simulink model "stewartplatform"  (R2019b)
settings: Solver=VariableStepAuto  StartTime=0.0  StopTime=34  RelTol=1e-3
model workspace (MAT data in the model file):
  AL = [69.992  30  41.1926948051; 60.9767621135  45.6148500617  41.1926948051; -60.9767621135  45.6148500617  41.1926948051; -69.992  30  41.1926948051; -9.01523788647  -75.6148500617  41.1926948051; 9.01523788647  -75.6148500617  41.1926948051]
  Alpha = [0.526894789881 2.61469786371 0.526894789881 2.61469786371 0.526894789881 2.61469786371]
  Alpha_ = [0.52689 2.6147 0.52689 2.6147 0.52689 2.6147]
  R = 71.492
  d = 58
  l = 1.5
  out = Simulink.SimulationOutput
  out.Data.tout = [0 3.15544362088e-30 0.00033203125 0.000660386534642 0.0011111273553 0.00167537750091 0.00236799304842 0.00321669373171 0.00427694118459 0.00567437280072 0.00710195631181 0.00848302964009 ... (1098 elements, 1098x1)]
  out.Metadata = Simulink.SimulationMetadata
  out.Metadata.ModelInfo.ModelName = 'stuartplatform'
  out.Metadata.ModelInfo.ModelVersion = '1.33'
  out.Metadata.ModelInfo.ModelFilePath = 'C:\DEV\stuartplatform\stuartplatform.slx'
  out.Metadata.ModelInfo.UserID = 'SMART PC'
  out.Metadata.ModelInfo.MachineName = 'ROBO'
  out.Metadata.ModelInfo.Platform = 'PCWIN64'
  out.Metadata.ModelInfo.ModelStructuralChecksum = [1978751953; 3150765780; 824817462; 4061112088]
  out.Metadata.ModelInfo.SimulationMode = 'normal'
  out.Metadata.ModelInfo.StartTime = 0
  out.Metadata.ModelInfo.StopTime = 1.68393954484
  out.Metadata.ModelInfo.SolverInfo.Type = 'Variable-Step'
  out.Metadata.ModelInfo.SolverInfo.Solver = 'ode45'
  out.Metadata.ModelInfo.SolverInfo.MaxStepSize = 0.68
  out.Metadata.ModelInfo.SimulinkVersion.Name = 'Simulink'
  out.Metadata.ModelInfo.SimulinkVersion.Version = '10.0'
  out.Metadata.ModelInfo.SimulinkVersion.Release = '(R2019b)'
  out.Metadata.ModelInfo.SimulinkVersion.Date = '18-Jul-2019'
  out.Metadata.ModelInfo.LoggingInfo.LoggingToFile = 'off'
  out.Metadata.TimingInfo.WallClockTimestampStart = '2020-06-21 19:02:22'
  out.Metadata.TimingInfo.WallClockTimestampStop = '2020-06-21 19:02:29'
  out.Metadata.TimingInfo.InitializationElapsedWallTime = 2.0463991
  out.Metadata.TimingInfo.ExecutionElapsedWallTime = 4.395282
  out.Metadata.TimingInfo.TerminationElapsedWallTime = 0.0061196
  out.Metadata.TimingInfo.TotalElapsedWallTime = 6.4478007
  out.Metadata.ExecutionInfo.StopEvent = 'StopCommand'
  out.Metadata.ExecutionInfo.StopEventSource = []
  out.Metadata.ExecutionInfo.StopEventDescription = 'Stop command issued at time 1.68394'
  out.Metadata.ExecutionInfo.ErrorDiagnostic = []
  out.Metadata.ExecutionInfo.WarningDiagnostics = struct([])
  out.Metadata.AppInfo = struct()
  p = 25
  q = 5.79
  r = 17.5
  rotangle = 1.0471975512
  smbData.shaping_wheels.Left.RigidTransform.angles = [1.57079632679 0.523598775598 0]
  smbData.shaping_wheels.Left.RigidTransform.ID = ''
  smbData.side_servo_SG90(1).Left.RigidTransform.angles = [1.57079632679 0 -1.0471975512]
  smbData.side_servo_SG90(1).Left.RigidTransform.translation = [59.315811956; 45.5; 34.246]
  smbData.side_servo_SG90(1).Left.RigidTransform.ID = ''
  smbData.side_servo_SG90(2).Left.RigidTransform.angles = [1.57079632679 0 -2.09439510239]
  smbData.side_servo_SG90(2).Left.RigidTransform.translation = [59.315811956; 45.5; -34.246]
  smbData.side_servo_SG90(2).Left.RigidTransform.ID = ''
  smbData.side_servo_SG90(3).Left.RigidTransform.angles = [1.57079632679 0 -3.14159265359]
  smbData.side_servo_SG90(3).Left.RigidTransform.translation = [8.38785085672e-15; 45.5; -68.492]
  smbData.side_servo_SG90(3).Left.RigidTransform.ID = ''
  smbData.side_servo_SG90(4).Left.RigidTransform.angles = [1.57079632679 0 -4.18879020479]
  smbData.side_servo_SG90(4).Left.RigidTransform.translation = [-59.315811956; 45.5; -34.246]
  smbData.side_servo_SG90(4).Left.RigidTransform.ID = ''
  smbData.side_servo_SG90(5).Left.RigidTransform.angles = [1.57079632679 0 -5.23598775598]
  smbData.side_servo_SG90(5).Left.RigidTransform.translation = [-59.315811956; 45.5; 34.246]
  smbData.side_servo_SG90(5).Left.RigidTransform.ID = ''
  smbData.side_servo_SG90(6).Left.RigidTransform.angles = [1.57079632679 0 -6.28318530718]
  smbData.side_servo_SG90(6).Left.RigidTransform.translation = [-1.67757017134e-14; 45.5; 68.492]
  smbData.side_servo_SG90(6).Left.RigidTransform.ID = ''
  smbData.servo_SG90(1).Left.RigidTransform.angles = [0 0 0]
  smbData.servo_SG90(1).Right.RigidTransform.angles = [-1.57079632679 0 0]
  smbData.servo_SG90(1).Right.RigidTransform.translation = [-5.79; 11.5; 0]
  smbData.servo_SG90(1).Right.RigidTransform.ID = ''
  smbData.servo_SG90(2).Left.RigidTransform.angles = [0 3.14159265359 0]
  smbData.servo_SG90(2).Right.RigidTransform.angles = [-1.57079632679 0 3.14159265359]
  smbData.servo_SG90(2).Right.RigidTransform.translation = [-5.79; 11.5; 0]
  smbData.servo_SG90(2).Right.RigidTransform.ID = ''
  smbData.servo_SG90(3).Left.RigidTransform.angles = [0 6.28318530718 0]
  smbData.servo_SG90(3).Right.RigidTransform.angles = [-1.57079632679 0 6.28318530718]
  smbData.servo_SG90(3).Right.RigidTransform.translation = [-5.79; 11.5; 0]
  smbData.servo_SG90(3).Right.RigidTransform.ID = ''
  smbData.servo_SG90(4).Left.RigidTransform.angles = [0 9.42477796077 0]
  smbData.servo_SG90(4).Right.RigidTransform.angles = [-1.57079632679 0 9.42477796077]
  smbData.servo_SG90(4).Right.RigidTransform.translation = [-5.79; 11.5; 0]
  smbData.servo_SG90(4).Right.RigidTransform.ID = ''
  smbData.servo_SG90(5).Left.RigidTransform.angles = [0 12.5663706144 0]
  smbData.servo_SG90(5).Right.RigidTransform.angles = [-1.57079632679 0 12.5663706144]
  smbData.servo_SG90(5).Right.RigidTransform.translation = [-5.79; 11.5; 0]
  smbData.servo_SG90(5).Right.RigidTransform.ID = ''
  smbData.servo_SG90(6).Left.RigidTransform.angles = [0 15.7079632679 0]
  smbData.servo_SG90(6).Right.RigidTransform.angles = [-1.57079632679 0 15.7079632679]
  smbData.servo_SG90(6).Right.RigidTransform.translation = [-5.79; 11.5; 0]
  smbData.servo_SG90(6).Right.RigidTransform.ID = ''
  smbData.link_active(1).Left.RigidTransform.angles = [1.57079632679 0 0]
  smbData.link_active(1).Left.RigidTransform.ID = ''
  smbData.link_active(1).Right.RigidTransform.angles = [1.57079632679 0 3.14159265359]
  smbData.link_active(1).Right.RigidTransform.translation = [-15.1842023169; 16.5; 0]
  smbData.link_active(1).Right.RigidTransform.ID = ''
  smbData.link_active(2).Left.RigidTransform.angles = [1.57079632679 0 0]
  smbData.link_active(2).Left.RigidTransform.ID = ''
  smbData.link_active(2).Right.RigidTransform.angles = [1.57079632679 0 6.28318530718]
  smbData.link_active(2).Right.RigidTransform.translation = [-15.1842023169; 16.5; 0]
  smbData.link_active(2).Right.RigidTransform.ID = ''
  smbData.link_active(3).Left.RigidTransform.angles = [1.57079632679 0 0]
  smbData.link_active(3).Left.RigidTransform.ID = ''
  smbData.link_active(3).Right.RigidTransform.angles = [1.57079632679 0 9.42477796077]
  smbData.link_active(3).Right.RigidTransform.translation = [-15.1842023169; 16.5; 0]
  smbData.link_active(3).Right.RigidTransform.ID = ''
  smbData.link_active(4).Left.RigidTransform.angles = [1.57079632679 0 0]
  smbData.link_active(4).Left.RigidTransform.ID = ''
  smbData.link_active(4).Right.RigidTransform.angles = [1.57079632679 0 12.5663706144]
  smbData.link_active(4).Right.RigidTransform.translation = [-15.1842023169; 16.5; 0]
  smbData.link_active(4).Right.RigidTransform.ID = ''
  smbData.link_active(5).Left.RigidTransform.angles = [1.57079632679 0 0]
  smbData.link_active(5).Left.RigidTransform.ID = ''
  smbData.link_active(5).Right.RigidTransform.angles = [1.57079632679 0 15.7079632679]
  smbData.link_active(5).Right.RigidTransform.translation = [-15.1842023169; 16.5; 0]
  smbData.link_active(5).Right.RigidTransform.ID = ''
  smbData.link_active(6).Left.RigidTransform.angles = [1.57079632679 0 0]
  smbData.link_active(6).Left.RigidTransform.ID = ''
  smbData.link_active(6).Right.RigidTransform.angles = [1.57079632679 0 18.8495559215]
  smbData.link_active(6).Right.RigidTransform.translation = [-15.1842023169; 16.5; 0]
  smbData.link_active(6).Right.RigidTransform.ID = ''
  smbData.joint_universal_between_axises_30 = [0 8.7 0]
  smbData.joint_universal_between_axises_15 = [0 8.7 0]
  smbData.joint_universal_30(1).Right.RigidTransform.angles = [0 0 0.520302761315]
  smbData.joint_universal_30(2).Right.RigidTransform.angles = [0 0 -0.520302761315]
  smbData.joint_universal_30(3).Right.RigidTransform.angles = [0 0 0.520302761315]
  smbData.joint_universal_30(4).Right.RigidTransform.angles = [0 0 -0.520302761315]
  smbData.joint_universal_30(5).Right.RigidTransform.angles = [0 0 0.520302761315]
  smbData.joint_universal_30(6).Right.RigidTransform.angles = [0 0 -0.520302761315]
  smbData.joint_universal_cube(1).Left.RigidTransform.angles = [0 0 -0.0054062780322]
  smbData.joint_universal_cube(1).Right.RigidTransform.angles = [0 1.57079632679 0.474503156818]
  smbData.joint_universal_cube(2).Left.RigidTransform.angles = [0 0 0.00540627803224]
  smbData.joint_universal_cube(2).Right.RigidTransform.angles = [0 1.57079632679 0.474503156818]
  smbData.joint_universal_cube(3).Left.RigidTransform.angles = [0 0 -0.0054062780322]
  smbData.joint_universal_cube(3).Right.RigidTransform.angles = [0 1.57079632679 0.474503156818]
  smbData.joint_universal_cube(4).Left.RigidTransform.angles = [0 0 0.00540627803224]
  smbData.joint_universal_cube(4).Right.RigidTransform.angles = [0 1.57079632679 0.474503156818]
  smbData.joint_universal_cube(5).Left.RigidTransform.angles = [0 0 -0.0054062780322]
  smbData.joint_universal_cube(5).Right.RigidTransform.angles = [0 1.57079632679 0.474503156818]
  smbData.joint_universal_cube(6).Left.RigidTransform.angles = [0 0 0.0054062780322]
  smbData.joint_universal_cube(6).Right.RigidTransform.angles = [0 1.57079632679 0.474503156818]
  smbData.joint_universal_15(1).Left.RigidTransform.angles = [0 0 -3.14159265359]
  smbData.joint_universal_15(1).Right.RigidTransform.angles = [3.14159265359 3.14159265359 0]
  smbData.joint_universal_15(2).Left.RigidTransform.angles = [0 0 -3.14159265359]
  smbData.joint_universal_15(2).Right.RigidTransform.angles = [3.14159265359 3.14159265359 0]
  smbData.joint_universal_15(3).Left.RigidTransform.angles = [0 0 -3.14159265359]
  smbData.joint_universal_15(3).Right.RigidTransform.angles = [3.14159265359 3.14159265359 0]
  smbData.joint_universal_15(4).Left.RigidTransform.angles = [0 0 -3.14159265359]
  smbData.joint_universal_15(4).Right.RigidTransform.angles = [3.14159265359 3.14159265359 0]
  smbData.joint_universal_15(5).Left.RigidTransform.angles = [0 0 -3.14159265359]
  smbData.joint_universal_15(5).Right.RigidTransform.angles = [3.14159265359 3.14159265359 0]
  smbData.joint_universal_15(6).Left.RigidTransform.angles = [0 0 -3.14159265359]
  smbData.joint_universal_15(6).Right.RigidTransform.angles = [3.14159265359 3.14159265359 0]
  smbData.joint_spherical(1).Left.RigidTransform.translation = [0 49.3 0]
  smbData.joint_spherical(1).Right.RigidTransform.translation = [69.992 41.1926948051 30]
  smbData.joint_spherical(2).Left.RigidTransform.translation = [0 49.3 0]
  smbData.joint_spherical(2).Right.RigidTransform.translation = [60.9767621135 41.1926948051 45.6148500617]
  smbData.joint_spherical(3).Left.RigidTransform.translation = [0 49.3 0]
  smbData.joint_spherical(3).Right.RigidTransform.translation = [-60.9767621135 41.1926948051 45.6148500617]
  smbData.joint_spherical(4).Left.RigidTransform.translation = [0 49.3 0]
  smbData.joint_spherical(4).Right.RigidTransform.translation = [-69.992 41.1926948051 30]
  smbData.joint_spherical(5).Left.RigidTransform.translation = [0 49.3 0]
  smbData.joint_spherical(5).Right.RigidTransform.translation = [-9.01523788647 41.1926948051 -75.6148500617]
  smbData.joint_spherical(6).Left.RigidTransform.translation = [0 49.3 0]
  smbData.joint_spherical(6).Right.RigidTransform.translation = [9.01523788647 41.1926948051 -75.6148500617]
  smbData.magnet(1).Left.RigidTransform.angles = [3.14159265359 0 0]
  smbData.magnet(1).Left.RigidTransform.translation = [0 6.2 0]
  smbData.magnet(2).Left.RigidTransform.angles = [3.14159265359 0 0]
  smbData.magnet(2).Left.RigidTransform.translation = [0 6.2 0]
  smbData.magnet(3).Left.RigidTransform.angles = [3.14159265359 0 0]
  smbData.magnet(3).Left.RigidTransform.translation = [0 6.2 0]
  smbData.magnet(4).Left.RigidTransform.angles = [3.14159265359 0 0]
  smbData.magnet(4).Left.RigidTransform.translation = [0 6.2 0]
  smbData.magnet(5).Left.RigidTransform.angles = [3.14159265359 0 0]
  smbData.magnet(5).Left.RigidTransform.translation = [0 6.2 0]
  smbData.magnet(6).Left.RigidTransform.angles = [3.14159265359 0 0]
  smbData.magnet(6).Left.RigidTransform.translation = [0 6.2 0]
  smbData.magnet_mount(1).Left.RigidTransform.angles = [0 0 0]
  smbData.magnet_mount(1).Left.RigidTransform.translation = [30 -7.2 69.992]
  smbData.magnet_mount(2).Left.RigidTransform.angles = [0 4.18879020479 0]
  smbData.magnet_mount(2).Left.RigidTransform.translation = [45.6148500617 -7.2 60.9767621135]
  smbData.magnet_mount(3).Left.RigidTransform.angles = [0 2.09439510239 0]
  smbData.magnet_mount(3).Left.RigidTransform.translation = [45.6148500617 -7.2 -60.9767621135]
  smbData.magnet_mount(4).Left.RigidTransform.angles = [0 6.28318530718 0]
  smbData.magnet_mount(4).Left.RigidTransform.translation = [30 -7.2 -69.992]
  smbData.magnet_mount(5).Left.RigidTransform.angles = [0 4.18879020479 0]
  smbData.magnet_mount(5).Left.RigidTransform.translation = [-75.6148500617 -7.2 -9.01523788647]
  smbData.magnet_mount(6).Left.RigidTransform.angles = [0 8.37758040957 0]
  smbData.magnet_mount(6).Left.RigidTransform.translation = [-75.6148500617 -7.2 9.01523788647]
  smbData.shaping_cover.Left.RigidTransform.angles = [1.57079632679 1.57079632679 0]
  smbData.shaping_cover.Left.RigidTransform.translation = [0 0 93.8626948051]
  smbData.shaping_cover.Left.RigidTransform.ID = ''
  smiData.shaping_wheels.mass = 0.0473643472469
  smiData.shaping_wheels.CoM = [0.00904094620934 1.50000000001 0.00637237485496]
  smiData.shaping_wheels.MoI = [70.380971606 150.089921057 79.7799959522]
  smiData.shaping_wheels.PoI = [0 -0.00787183150838 9.1710814623e-09]
  smiData.shaping_wheels.color = [1 0.4 0]
  smiData.shaping_wheels.opacity = 1
  smiData.shaping_wheels.ID = 'solid_shaping_wheels'
  smiData.shaping_ring.mass = 0.0385673660956
  smiData.shaping_ring.CoM = [0.0102207277286 2.00000000002 0.0148576027735]
  smiData.shaping_ring.MoI = [85.1814256802 170.315961217 85.2373818669]
  smiData.shaping_ring.PoI = [0 4.14524405806e-05 0]
  smiData.shaping_ring.color = [1 0.4 0]
  smiData.shaping_ring.opacity = 1
  smiData.shaping_ring.ID = 'solid_shaping_ring'
  smiData.joint_spherical.mass = 0.00598048800238
  smiData.joint_spherical.CoM = [0 16.7435459237 0]
  smiData.joint_spherical.MoI = [0.415501873425 0.0335614179001 0.415501873425]
  smiData.joint_spherical.PoI = [0.5 0.5 0.5]
  smiData.joint_spherical.color = [0.647058823529 0.619607843137 0.588235294118]
  smiData.joint_spherical.opacity = 1
  smiData.joint_spherical.ID = 'solid_joint_spherical_ball'
  smiData.side_servo_SG90.mass = 0.107401268683
  smiData.side_servo_SG90.CoM = [0.0100070028027 1.5 0.841284974509]
  smiData.side_servo_SG90.MoI = [36.4001993772 95.7087158602 59.4696185764]
  smiData.side_servo_SG90.PoI = [0 2.00251948913 0]
  smiData.side_servo_SG90.color = [1 0.4 0]
  smiData.side_servo_SG90.opacity = 1
  smiData.side_servo_SG90.ID = 'solid_side_servo_SG90'
  smiData.servo_sg90.mass = 0.00720704423786
  smiData.servo_sg90.CoM = [3.9865723068 -3.90328838164 9.80930800299e-08]
  smiData.servo_sg90.MoI = [0.466621426291 0.439244146793 0.731122278609]
  smiData.servo_sg90.PoI = [5.31816444263e-09 -4.96226215662e-08 0.0304040962781]
  smiData.servo_sg90.color = [0 0.2 1]
  smiData.servo_sg90.opacity = 1
  smiData.servo_sg90.ID = 'solid_servo_sg90'
  smiData.link_active_servomotion.mass = 0.0342098482698
  smiData.link_active_servomotion.CoM = [-10.0371053389 9.47462283796 -4.16922193987e-06]
  smiData.link_active_servomotion.MoI = [1.60054780115 2.26600734555 3.11405237421]
  smiData.link_active_servomotion.PoI = [5.2454163719e-07 1.42332906188e-06 0.261259593595]
  smiData.link_active_servomotion.color = [0.8 0.8 1]
  smiData.link_active_servomotion.opacity = 1
  smiData.link_active_servomotion.ID = 'solid_link_active_servomotion'
  smiData.joint_universal_30.mass = 0.00272196304974
  smiData.joint_universal_30.CoM = [6.19132995267e-05 4.11309808179 0.205474734378]
  smiData.joint_universal_30.MoI = [0.0492670374434 0.0334718549392 0.0423742684915]
  smiData.joint_universal_30.PoI = [0.000875816941094 -7.13748194627e-07 5.39567191258e-07]
  smiData.joint_universal_30.color = [0.647058823529 0.619607843137 0.588235294118]
  smiData.joint_universal_30.opacity = 1
  smiData.joint_universal_30.ID = 'solid_joint_universal_30'
  smiData.joint_universal_15.mass = 0.00283940186846
  smiData.joint_universal_15.CoM = [6.93872966997e-05 4.41865064988 0.19570305708]
  smiData.joint_universal_15.MoI = [0.0571401143275 0.035195609637 0.0486824772277]
  smiData.joint_universal_15.PoI = [0.00107238150077 -6.81084569699e-07 3.94146475722e-07]
  smiData.joint_universal_15.color = [0.647058823529 0.619607843137 0.588235294118]
  smiData.joint_universal_15.opacity = 1
  smiData.joint_universal_15.ID = 'solid_joint_universal_'
  smiData.joint_universal_cube.mass = 0.00129650759707
  smiData.joint_universal_cube.CoM = [-3.24129379478e-07 2.999999997 2.52027313647e-06]
  smiData.joint_universal_cube.MoI = [0.00869808529259 0.00848435534744 0.00929045529439]
  smiData.joint_universal_cube.PoI = [0 0 3.30706805855e-09]
  smiData.joint_universal_cube.color = [0.647058823529 0.619607843137 0.588235294118]
  smiData.joint_universal_cube.opacity = 1
  smiData.joint_universal_cube.ID = 'solid_joint_universal_cube'
  smiData.link_passive.mass = 0.00151035349225
  smiData.link_passive.CoM = [-2.7216183763e-06 -9.10785085243 0.0307676189295]
  smiData.link_passive.MoI = [0.169227176143 0.0195448717423 0.169460532499]
  smiData.link_passive.PoI = [-0.000637032298741 -1.63350578781e-08 5.1687228076e-08]
  smiData.link_passive.color = [0.6 0 0]
  smiData.link_passive.opacity = 1
  smiData.link_passive.ID = 'solid_link_passive'
  smiData.magnet.mass = 0.00143035205498
  smiData.magnet.CoM = [0 1.37066806046 0]
  smiData.magnet.MoI = [0.0116973776756 0.0214424284656 0.0116973776756]
  smiData.magnet.PoI = [0 0 0]
  smiData.magnet.color = [0.1 0.1 0.1]
  smiData.magnet.opacity = 1
  smiData.magnet.ID = 'solid_magnet'
  smiData.magnet_mount.mass = 0.00778165476871
  smiData.magnet_mount.CoM = [9.26571540214 52.0843662176 0]
  smiData.magnet_mount.MoI = [0.0882337997564 0.667327214154 0.624985588151]
  smiData.magnet_mount.PoI = [0 8.0383612392e-09 -0.00250850026421]
  smiData.magnet_mount.color = [0.9 0.9 0.9]
  smiData.magnet_mount.opacity = 1
  smiData.magnet_mount.ID = 'solid_magnet_mount'
  smiData.shaping_cover.mass = 0.18
  smiData.shaping_cover.CoM = [0.0262084599856 1.50000000001 -0.0195559891106]
  smiData.shaping_cover.MoI = [82.9846897967 165.937709417 83.0369065281]
  smiData.shaping_cover.PoI = [0 -0.00356804218787 0]
  smiData.shaping_cover.color = [0.5 0.5 0.5]
  smiData.shaping_cover.opacity = 0.5
  smiData.shaping_cover.ID = 'solid_shaping_cover'
undefined symbols (not defined in the file): X, Y, Z
libraries: sm_lib x167, nesl_utility x7, simulink x7, dspswit3 x2
(part 1 of 5)
settings Model: Creator=rprak  LastModifiedBy=SMART PC

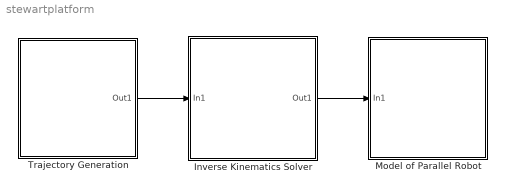
== system stewartplatform ==
  Inverse Kinematics Solver : Subsystem
      mask Display: image('icons\cheme.png'); % Use "Edit Image" on toolstrip to change.
  Model of Parallel Robot : Subsystem
      mask Display: image('icons\stuartplatformicon.png'); % Use "Edit Image" on toolstrip to change.
  Trajectory Generation : Subsystem
      mask Display: image('icons\wave_angles.png'); % Use "Edit Image" on toolstrip to change.
  wires:
  Trajectory Generation/1(Out1) -> Inverse Kinematics Solver/1(In1)
  Inverse Kinematics Solver/1(Out1) -> Model of Parallel Robot/1(In1)

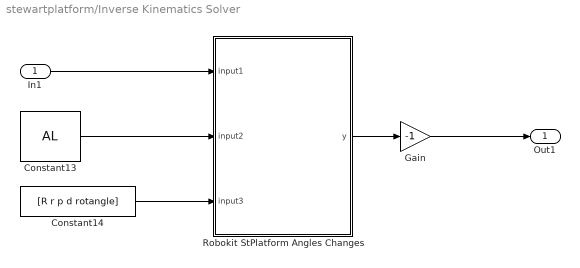
== system stewartplatform/Inverse Kinematics Solver ==
  In1 : Inport
  Constant13 : Constant  Value=AL
  Constant14 : Constant  Value=[R r p d rotangle]
  Gain : Gain  Gain=-1
  Robokit StPlatform Angles Changes : MATLAB Function  TreatAsAtomicUnit=on
  Out1 : Outport
  wires:
  Constant13/1 -> Robokit StPlatform Angles Changes/2(input2)
  Robokit StPlatform Angles Changes/1(y) -> Gain/1
  Constant14/1 -> Robokit StPlatform Angles Changes/3(input3)
  In1/1 -> Robokit StPlatform Angles Changes/1(input1)
  Gain/1 -> Out1/1

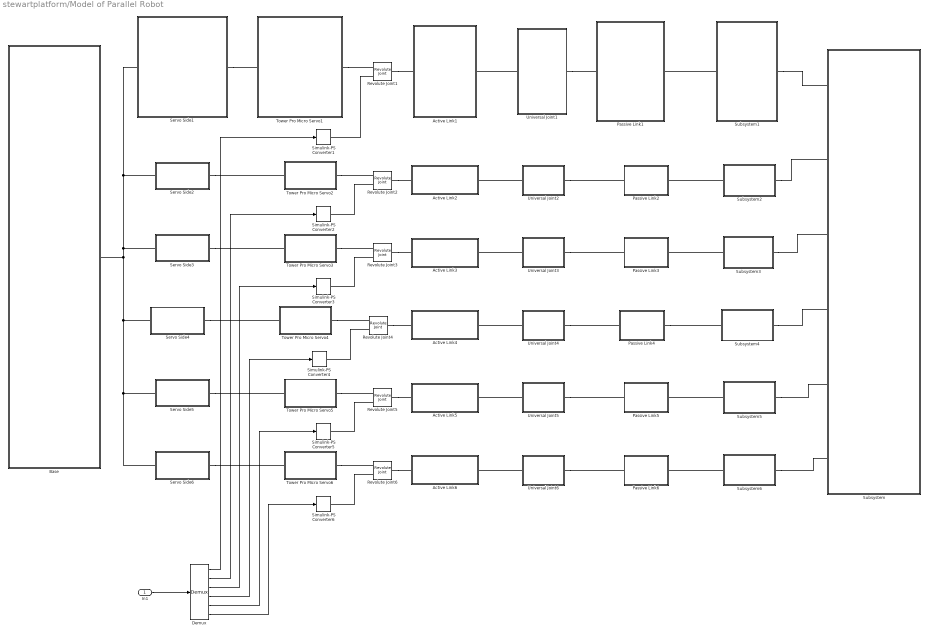
== system stewartplatform/Model of Parallel Robot ==
  In1 : Inport
  Active Link1 : Subsystem
      mask Display: image('icons\solid_chain_active.png'); % Use "Edit Image" on toolstrip to change.
  Active Link2 : Subsystem
  Active Link3 : Subsystem
  Active Link4 : Subsystem
  Active Link5 : Subsystem
  Active Link6 : Subsystem
  Base : Subsystem
      mask Display: image('C:\DEV\stuartplatform\icons\solid_base.png'); % Use "Edit Image" on toolstrip to change.
  Demux : Demux  Outputs=6
  Passive Link1 : Subsystem
      mask Display: image('icons\solid_chain_passive.png'); % Use "Edit Image" on toolstrip to change.
  Passive Link2 : Subsystem
  Passive Link3 : Subsystem
  Passive Link4 : Subsystem
  Passive Link5 : Subsystem
  Passive Link6 : Subsystem
  Revolute Joint{1..6} (6 alike) : sm_lib/Joints/Revolute Joint  JointMode=Normal  SenseConstraintForce=off  SenseConstraintForceX=off  SenseConstraintForceY=off  SenseConstraintForceZ=off  SenseConstraintTorque=off  SenseConstraintTorqueX=off  SenseConstraintTorqueY=off  SenseConstraintTorqueZ=off  SenseTotalForce=off  SenseTotalForceX=off  SenseTotalForceY=off  SenseTotalForceZ=off  SenseTotalTorque=off  SenseTotalTorqueX=off  SenseTotalTorqueY=off  SenseTotalTorqueZ=off  CompositeWrenchDir=FollowerOnBase  CompositeWrenchFrame=BaseFrame  EquilibriumPosition=0  EquilibriumPositionUnits=rad  SpringStiffness=0  SpringStiffnessUnits=N*m/deg  DampingCoefficient=0  DampingCoefficientUnits=N*m/(deg/s)  TorqueActuationMode=ComputedTorque  MotionActuationMode=InputMotion  SensePosition=off  SenseVelocity=off  SenseAcceleration=off  SenseTorqueForce=off  SenseLowerLimitTorqueForce=off  SenseUpperLimitTorqueForce=off  LowerLimitSpecify=off  LowerLimitBound=-90  LowerLimitBoundUnits=deg  LowerLimitStiffness=1e4  LowerLimitStiffnessUnits=N*m/deg  LowerLimitDamping=10  LowerLimitDampingUnits=N*m/(deg/s)  LowerLimitTransitionRegionWidth=0.1  LowerLimitTransitionRegionWidthUnits=deg  UpperLimitSpecify=off  UpperLimitBound=90  UpperLimitBoundUnits=deg  UpperLimitStiffness=1e4  UpperLimitStiffnessUnits=N*m/deg  UpperLimitDamping=10  UpperLimitDampingUnits=N*m/(deg/s)  UpperLimitTransitionRegionWidth=0.1  UpperLimitTransitionRegionWidthUnits=deg  PositionTargetSpecify=on  PositionTargetPriority=High  PositionTargetValue=0  PositionTargetValueUnits=rad  VelocityTargetSpecify=off  VelocityTargetPriority=High  VelocityTargetValue=1  VelocityTargetValueUnits=rad/s
  Servo Side1 : Subsystem
      mask Display: image('C:\DEV\stuartplatform\icons\solid_side.png'); % Use "Edit Image" on toolstrip to change.
  Servo Side2 : Subsystem
  Servo Side3 : Subsystem
  Servo Side4 : Subsystem
  Servo Side5 : Subsystem
  Servo Side6 : Subsystem
  Simulink-PS Converter{1..6} (6 alike) : nesl_utility/Simulink-PS Converter  PhysicalDomain=network_engine_domain  SubClassName=ps_input  LeftPortType=input  RightPortType=output  PseudoPeriodic=off  Frequencies=[]  NoiseDistribution=none  NoiseParameters=[]  Unit=rad  AffineConversion=off  FilteringAndDerivatives=filter  SimscapeFilterOrder=2  InputFilterTimeConstant=0.001  UdotUserProvided=0
  Subsystem : Subsystem
      mask Display: image('icons\solid_cover.png'); % Use "Edit Image" on toolstrip to change.
  Subsystem1 : Subsystem
      mask Display: image('icons\solid_magnet.png'); % Use "Edit Image" on toolstrip to change.
  Subsystem2 : Subsystem
  Subsystem3 : Subsystem
  Subsystem4 : Subsystem
  Subsystem5 : Subsystem
  Subsystem6 : Subsystem
  Tower Pro Micro Servo1 : Subsystem
      mask Display: image('icons\solid_motor.png'); % Use "Edit Image" on toolstrip to change.
  Tower Pro Micro Servo2 : Subsystem
  Tower Pro Micro Servo3 : Subsystem
  Tower Pro Micro Servo4 : Subsystem
  Tower Pro Micro Servo5 : Subsystem
  Tower Pro Micro Servo6 : Subsystem
  Universal Joint1 : Subsystem
      mask Display: image('icons\solid_joint_universal.png'); % Use "Edit Image" on toolstrip to change.
  Universal Joint2 : Subsystem
  Universal Joint3 : Subsystem
  Universal Joint4 : Subsystem
  Universal Joint5 : Subsystem
  Universal Joint6 : Subsystem
  wires:
  Demux/3 -> Simulink-PS Converter3/1
  Demux/5 -> Simulink-PS Converter5/1
  In1/1 -> Demux/1
  Demux/4 -> Simulink-PS Converter4/1
  Demux/2 -> Simulink-PS Converter2/1
  Demux/1 -> Simulink-PS Converter1/1
  Demux/6 -> Simulink-PS Converter6/1
  connections:
  Servo Side4/RConn1 -- Tower Pro Micro Servo4/LConn1
  Revolute Joint5/LConn2 -- Simulink-PS Converter5/RConn1
  Revolute Joint1/RConn1 -- Active Link1/LConn1
  Universal Joint4/RConn1 -- Passive Link4/LConn1
  Revolute Joint6/RConn1 -- Active Link6/LConn1
  Universal Joint6/LConn1 -- Active Link6/RConn1
  Tower Pro Micro Servo3/RConn1 -- Revolute Joint3/LConn1
  Universal Joint5/LConn1 -- Active Link5/RConn1
  Base/RConn1 -- Servo Side5/LConn1 -- Servo Side6/LConn1 -- Servo Side4/LConn1 -- Servo Side2/LConn1 -- Servo Side1/LConn1 -- Servo Side3/LConn1
  Revolute Joint2/LConn2 -- Simulink-PS Converter2/RConn1
  Universal Joint4/LConn1 -- Active Link4/RConn1
  Universal Joint1/RConn1 -- Passive Link1/LConn1
  Universal Joint5/RConn1 -- Passive Link5/LConn1
  Revolute Joint4/LConn2 -- Simulink-PS Converter4/RConn1
  Tower Pro Micro Servo2/RConn1 -- Revolute Joint2/LConn1
  Tower Pro Micro Servo1/RConn1 -- Revolute Joint1/LConn1
  Universal Joint2/RConn1 -- Passive Link2/LConn1
  Universal Joint1/LConn1 -- Active Link1/RConn1
  Universal Joint6/RConn1 -- Passive Link6/LConn1
  Servo Side1/RConn1 -- Tower Pro Micro Servo1/LConn1
  Servo Side6/RConn1 -- Tower Pro Micro Servo6/LConn1
  Servo Side2/RConn1 -- Tower Pro Micro Servo2/LConn1
  Tower Pro Micro Servo6/RConn1 -- Revolute Joint6/LConn1
  Revolute Joint1/LConn2 -- Simulink-PS Converter1/RConn1
  Revolute Joint3/RConn1 -- Active Link3/LConn1
  Servo Side3/RConn1 -- Tower Pro Micro Servo3/LConn1
  Revolute Joint4/RConn1 -- Active Link4/LConn1
  Universal Joint3/LConn1 -- Active Link3/RConn1
  Tower Pro Micro Servo5/RConn1 -- Revolute Joint5/LConn1
  Universal Joint2/LConn1 -- Active Link2/RConn1
  Revolute Joint2/RConn1 -- Active Link2/LConn1
  Servo Side5/RConn1 -- Tower Pro Micro Servo5/LConn1
  Universal Joint3/RConn1 -- Passive Link3/LConn1
  Revolute Joint6/LConn2 -- Simulink-PS Converter6/RConn1
  Revolute Joint3/LConn2 -- Simulink-PS Converter3/RConn1
  Tower Pro Micro Servo4/RConn1 -- Revolute Joint4/LConn1
  Revolute Joint5/RConn1 -- Active Link5/LConn1
  Subsystem6/LConn1 -- Passive Link6/RConn1
  Subsystem6/RConn1 -- Subsystem/LConn6
  Subsystem5/LConn1 -- Passive Link5/RConn1
  Subsystem5/RConn1 -- Subsystem/LConn5
  Passive Link4/RConn1 -- Subsystem4/LConn1
  Subsystem4/RConn1 -- Subsystem/LConn4
  Subsystem3/LConn1 -- Passive Link3/RConn1
  Subsystem3/RConn1 -- Subsystem/LConn3
  Subsystem2/LConn1 -- Passive Link2/RConn1
  Subsystem2/RConn1 -- Subsystem/LConn2
  Subsystem1/LConn1 -- Passive Link1/RConn1
  Subsystem1/RConn1 -- Subsystem/LConn1

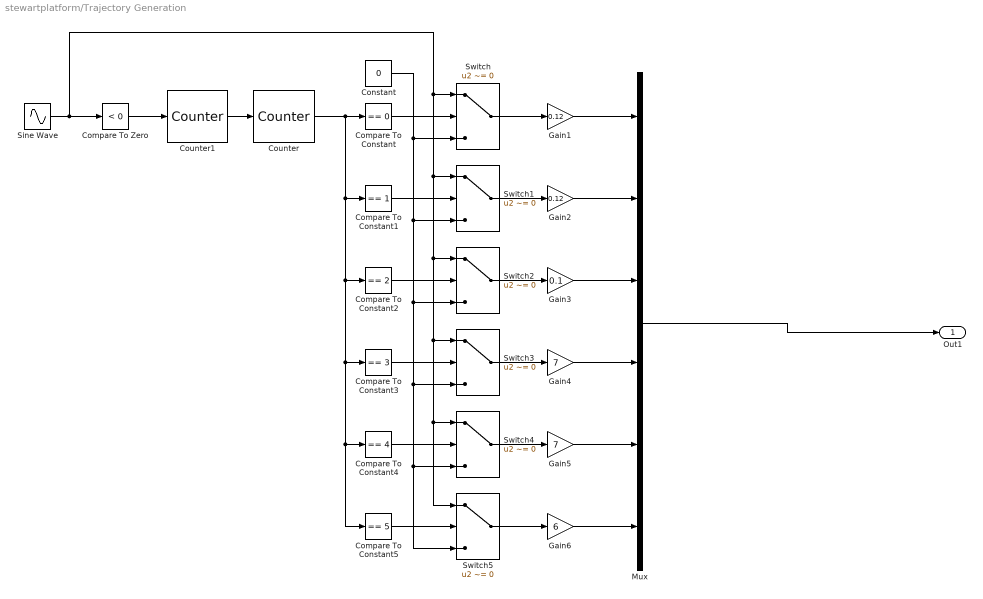
== system stewartplatform/Trajectory Generation ==
  Compare To Constant : simulink/Logic and Bit Operations/Compare To Constant  relop===  const=0  OutDataTypeStr=boolean
  Compare To Constant1 : simulink/Logic and Bit Operations/Compare To Constant  relop===  const=1  OutDataTypeStr=boolean
  Compare To Constant2 : simulink/Logic and Bit Operations/Compare To Constant  relop===  const=2  OutDataTypeStr=boolean
  Compare To Constant3 : simulink/Logic and Bit Operations/Compare To Constant  relop===  const=3  OutDataTypeStr=boolean
  Compare To Constant4 : simulink/Logic and Bit Operations/Compare To Constant  relop===  const=4  OutDataTypeStr=boolean
  Compare To Constant5 : simulink/Logic and Bit Operations/Compare To Constant  relop===  const=5  OutDataTypeStr=boolean
  Compare To Zero : simulink/Logic and Bit Operations/Compare To Zero  relop=<  OutDataTypeStr=boolean
  Constant : Constant  Value=0
  Counter : dspswit3/Counter  Direction=Up  CountEvent=Rising edge  CounterSize=User defined  MaxCount=5  InitialCount=0  Output=Count  HitValue=32  ResetInput=off  SamplesPerFrame=1  Ts=1  CntDtype=double  HitDtype=Logical
  Counter1 : dspswit3/Counter  Direction=Up  CountEvent=Rising edge  CounterSize=User defined  MaxCount=2  InitialCount=0  Output=Hit  HitValue=2  ResetInput=off  SamplesPerFrame=1  Ts=1  CntDtype=double  HitDtype=Logical
  Gain1 : Gain  Gain=0.12
  Gain2 : Gain  Gain=0.12
  Gain3 : Gain  Gain=0.1
  Gain4 : Gain  Gain=7
  Gain5 : Gain  Gain=7
  Gain6 : Gain  Gain=6
  Mux : Mux  Inputs=6
  Sine Wave : Sin  Frequency=3  SampleTime=0
  Switch{,1..5} (6 alike) : Switch  Criteria=u2 ~= 0
  Out1 : Outport
  wires:
  Gain2/1 -> Mux/2
  Counter/1 -> Compare To Constant1/1, Compare To Constant5/1, Compare To Constant4/1, Compare To Constant3/1, Compare To Constant2/1, Compare To Constant/1
  Mux/1 -> Out1/1
  Compare To Constant3/1 -> Switch3/2
  Switch5/1 -> Gain6/1
  Sine Wave/1 -> Compare To Zero/1, Switch5/1, Switch4/1, Switch3/1, Switch2/1, Switch1/1, Switch/1
  Gain1/1 -> Mux/1
  Gain6/1 -> Mux/6
  Compare To Constant/1 -> Switch/2
  Constant/1 -> Switch1/3, Switch2/3, Switch3/3, Switch4/3, Switch5/3, Switch/3
  Compare To Constant5/1 -> Switch5/2
  Switch/1 -> Gain1/1
  Switch1/1 -> Gain2/1
  Gain4/1 -> Mux/4
  Compare To Constant2/1 -> Switch2/2
  Gain3/1 -> Mux/3
  Compare To Constant4/1 -> Switch4/2
  Switch3/1 -> Gain4/1
  Gain5/1 -> Mux/5
  Switch4/1 -> Gain5/1
  Switch2/1 -> Gain3/1
  Compare To Zero/1 -> Counter1/1
  Counter1/1 -> Counter/1
  Compare To Constant1/1 -> Switch1/2

== system stewartplatform/Model of Parallel Robot/Active Link1 ==
  Rigid Transform : sm_lib/Frames and Transforms/Rigid Transform  TranslationMethod=None  TranslationStandardOffset=0  TranslationLengthUnit=m  TranslationStandardAxis=+Z  TranslationCartesianOffset=[0 0 0]  TranslationROffset=0  TranslationROffsetUnits=m  TranslationZOffset=0  TranslationZOffsetUnits=m  TranslationThetaOffset=0  TranslationThetaOffsetUnits=deg  RotationMethod=RotationSequence  RotationAngleUnits=deg  RotationStandardAxis=+Z  RotationAngle=0.0  RotationArbitraryAxis=[0 0 1]  FollAlignAxisA=+X  BaseAlignAxisA=+Y  FollAlignAxisB=+Y  BaseAlignAxisB=+Z  RotationSequenceAxes=FollowerAxes  RotationSequence=XYZ  RotationSequenceAngles=smbData.link_active(1).Left.RigidTransform.angles  RotationSequenceAnglesUnits=rad  RotationMatrix=[1 0 0; 0 1 0; 0 0 1]
  Rigid Transform5 : sm_lib/Frames and Transforms/Rigid Transform  TranslationMethod=Cartesian  TranslationStandardOffset=0  TranslationLengthUnit=mm  TranslationStandardAxis=+Z  TranslationCartesianOffset=smbData.link_active(1).Right.RigidTransform.translation  TranslationROffset=0  TranslationROffsetUnits=m  TranslationZOffset=0  TranslationZOffsetUnits=m  TranslationThetaOffset=0  TranslationThetaOffsetUnits=deg  RotationMethod=RotationSequence  RotationAngleUnits=deg  RotationStandardAxis=+X  RotationAngle=90.0  RotationArbitraryAxis=[0 0 1]  FollAlignAxisA=+X  BaseAlignAxisA=+Y  FollAlignAxisB=+Y  BaseAlignAxisB=+Z  RotationSequenceAxes=FollowerAxes  RotationSequence=XYZ  RotationSequenceAngles=smbData.link_active(1).Right.RigidTransform.angles  RotationSequenceAnglesUnits=rad  RotationMatrix=[1 0 0; 0 1 0; 0 0 1]
  link_active_servomotion : sm_lib/Body Elements/File Solid  ExtGeomFileName=meshes\link_active_servomotion.STEP  UnitType=FromFile  ExtGeomFileUnits=m  StepReaderType=HEX  ExportEntireGeometry=off  InertiaType=Custom  Mass=smiData.link_active_servomotion.mass  MassUnits=kg  CenterOfMass=smiData.link_active_servomotion.CoM  CenterOfMassUnits=m  MomentsOfInertia=smiData.link_active_servomotion.MoI  MomentsOfInertiaUnits=kg*m^2  ProductsOfInertia=smiData.link_active_servomotion.PoI  ProductsOfInertiaUnits=kg*m^2  BasedOnType=Density  Density=1000  DensityUnits=kg/m^3  DoExposeReferenceFrame=on  SerializedFrames=<Frames/>  GraphicType=FromGeometry  MarkerShape=Sphere  MarkerSize=10  GraphicVisPropType=SimpleVisualProperties  GraphicDiffuseColor=smiData.link_active_servomotion.color  GraphicSpecularColor=[0.5 0.5 0.5 1.0]  GraphicAmbientColor=[0.15 0.15 0.15 1.0]  GraphicEmissiveColor=[0.0 0.0 0.0 1.0]  GraphicShininess=75  GraphicOpacity=smiData.link_active_servomotion.opacity
  Conn1 : PMIOPort  Side=Left
  Conn2 : PMIOPort  Port=2  Side=Right
  connections:
  Rigid Transform5/LConn1 -- Rigid Transform/RConn1 -- link_active_servomotion/RConn1
  Rigid Transform/LConn1 -- Conn1/RConn1
  Conn2/RConn1 -- Rigid Transform5/RConn1

== system stewartplatform/Model of Parallel Robot/Active Link2 ==
  Rigid Transform : sm_lib/Frames and Transforms/Rigid Transform  TranslationMethod=None  TranslationStandardOffset=0  TranslationLengthUnit=m  TranslationStandardAxis=+Z  TranslationCartesianOffset=[0 0 0]  TranslationROffset=0  TranslationROffsetUnits=m  TranslationZOffset=0  TranslationZOffsetUnits=m  TranslationThetaOffset=0  TranslationThetaOffsetUnits=deg  RotationMethod=RotationSequence  RotationAngleUnits=deg  RotationStandardAxis=+Z  RotationAngle=0.0  RotationArbitraryAxis=[0 0 1]  FollAlignAxisA=+X  BaseAlignAxisA=+Y  FollAlignAxisB=+Y  BaseAlignAxisB=+Z  RotationSequenceAxes=FollowerAxes  RotationSequence=XYZ  RotationSequenceAngles=smbData.link_active(2).Left.RigidTransform.angles  RotationSequenceAnglesUnits=rad  RotationMatrix=[1 0 0; 0 1 0; 0 0 1]
  Rigid Transform5 : sm_lib/Frames and Transforms/Rigid Transform  TranslationMethod=Cartesian  TranslationStandardOffset=0  TranslationLengthUnit=mm  TranslationStandardAxis=+Z  TranslationCartesianOffset=smbData.link_active(2).Right.RigidTransform.translation  TranslationROffset=0  TranslationROffsetUnits=m  TranslationZOffset=0  TranslationZOffsetUnits=m  TranslationThetaOffset=0  TranslationThetaOffsetUnits=deg  RotationMethod=RotationSequence  RotationAngleUnits=deg  RotationStandardAxis=+X  RotationAngle=90.0  RotationArbitraryAxis=[0 0 1]  FollAlignAxisA=+X  BaseAlignAxisA=+Y  FollAlignAxisB=+Y  BaseAlignAxisB=+Z  RotationSequenceAxes=FollowerAxes  RotationSequence=XYZ  RotationSequenceAngles=smbData.link_active(2).Right.RigidTransform.angles  RotationSequenceAnglesUnits=rad  RotationMatrix=[1 0 0; 0 1 0; 0 0 1]
  link_active_servomotion : sm_lib/Body Elements/File Solid  ExtGeomFileName=meshes\link_active_servomotion.STEP  UnitType=FromFile  ExtGeomFileUnits=m  StepReaderType=HEX  ExportEntireGeometry=off  InertiaType=Custom  Mass=smiData.link_active_servomotion.mass  MassUnits=kg  CenterOfMass=smiData.link_active_servomotion.CoM  CenterOfMassUnits=m  MomentsOfInertia=smiData.link_active_servomotion.MoI  MomentsOfInertiaUnits=kg*m^2  ProductsOfInertia=smiData.link_active_servomotion.PoI  ProductsOfInertiaUnits=kg*m^2  BasedOnType=Density  Density=1000  DensityUnits=kg/m^3  DoExposeReferenceFrame=on  SerializedFrames=<Frames/>  GraphicType=FromGeometry  MarkerShape=Sphere  MarkerSize=10  GraphicVisPropType=SimpleVisualProperties  GraphicDiffuseColor=smiData.link_active_servomotion.color  GraphicSpecularColor=[0.5 0.5 0.5 1.0]  GraphicAmbientColor=[0.15 0.15 0.15 1.0]  GraphicEmissiveColor=[0.0 0.0 0.0 1.0]  GraphicShininess=75  GraphicOpacity=smiData.link_active_servomotion.opacity
  Conn1 : PMIOPort  Side=Left
  Conn2 : PMIOPort  Port=2  Side=Right
  connections:
  Rigid Transform5/LConn1 -- link_active_servomotion/RConn1 -- Rigid Transform/RConn1
  Rigid Transform/LConn1 -- Conn1/RConn1
  Conn2/RConn1 -- Rigid Transform5/RConn1

== system stewartplatform/Model of Parallel Robot/Active Link3 ==
  Rigid Transform : sm_lib/Frames and Transforms/Rigid Transform  TranslationMethod=None  TranslationStandardOffset=0  TranslationLengthUnit=m  TranslationStandardAxis=+Z  TranslationCartesianOffset=[0 0 0]  TranslationROffset=0  TranslationROffsetUnits=m  TranslationZOffset=0  TranslationZOffsetUnits=m  TranslationThetaOffset=0  TranslationThetaOffsetUnits=deg  RotationMethod=RotationSequence  RotationAngleUnits=deg  RotationStandardAxis=+Z  RotationAngle=0.0  RotationArbitraryAxis=[0 0 1]  FollAlignAxisA=+X  BaseAlignAxisA=+Y  FollAlignAxisB=+Y  BaseAlignAxisB=+Z  RotationSequenceAxes=FollowerAxes  RotationSequence=XYZ  RotationSequenceAngles=smbData.link_active(3).Left.RigidTransform.angles  RotationSequenceAnglesUnits=rad  RotationMatrix=[1 0 0; 0 1 0; 0 0 1]
  Rigid Transform5 : sm_lib/Frames and Transforms/Rigid Transform  TranslationMethod=Cartesian  TranslationStandardOffset=0  TranslationLengthUnit=mm  TranslationStandardAxis=+Z  TranslationCartesianOffset=smbData.link_active(3).Right.RigidTransform.translation  TranslationROffset=0  TranslationROffsetUnits=m  TranslationZOffset=0  TranslationZOffsetUnits=m  TranslationThetaOffset=0  TranslationThetaOffsetUnits=deg  RotationMethod=RotationSequence  RotationAngleUnits=deg  RotationStandardAxis=+X  RotationAngle=90.0  RotationArbitraryAxis=[0 0 1]  FollAlignAxisA=+X  BaseAlignAxisA=+Y  FollAlignAxisB=+Y  BaseAlignAxisB=+Z  RotationSequenceAxes=FollowerAxes  RotationSequence=XYZ  RotationSequenceAngles=smbData.link_active(3).Right.RigidTransform.angles  RotationSequenceAnglesUnits=rad  RotationMatrix=[1 0 0; 0 1 0; 0 0 1]
  link_active_servomotion : sm_lib/Body Elements/File Solid  ExtGeomFileName=meshes\link_active_servomotion.STEP  UnitType=FromFile  ExtGeomFileUnits=m  StepReaderType=HEX  ExportEntireGeometry=off  InertiaType=Custom  Mass=smiData.link_active_servomotion.mass  MassUnits=kg  CenterOfMass=smiData.link_active_servomotion.CoM  CenterOfMassUnits=m  MomentsOfInertia=smiData.link_active_servomotion.MoI  MomentsOfInertiaUnits=kg*m^2  ProductsOfInertia=smiData.link_active_servomotion.PoI  ProductsOfInertiaUnits=kg*m^2  BasedOnType=Density  Density=1000  DensityUnits=kg/m^3  DoExposeReferenceFrame=on  SerializedFrames=<Frames/>  GraphicType=FromGeometry  MarkerShape=Sphere  MarkerSize=10  GraphicVisPropType=SimpleVisualProperties  GraphicDiffuseColor=smiData.link_active_servomotion.color  GraphicSpecularColor=[0.5 0.5 0.5 1.0]  GraphicAmbientColor=[0.15 0.15 0.15 1.0]  GraphicEmissiveColor=[0.0 0.0 0.0 1.0]  GraphicShininess=75  GraphicOpacity=smiData.link_active_servomotion.opacity
  Conn1 : PMIOPort  Side=Left
  Conn2 : PMIOPort  Port=2  Side=Right
  connections:
  Rigid Transform5/LConn1 -- Rigid Transform/RConn1 -- link_active_servomotion/RConn1
  Rigid Transform/LConn1 -- Conn1/RConn1
  Conn2/RConn1 -- Rigid Transform5/RConn1

== system stewartplatform/Model of Parallel Robot/Active Link4 ==
  Rigid Transform : sm_lib/Frames and Transforms/Rigid Transform  TranslationMethod=None  TranslationStandardOffset=0  TranslationLengthUnit=m  TranslationStandardAxis=+Z  TranslationCartesianOffset=[0 0 0]  TranslationROffset=0  TranslationROffsetUnits=m  TranslationZOffset=0  TranslationZOffsetUnits=m  TranslationThetaOffset=0  TranslationThetaOffsetUnits=deg  RotationMethod=RotationSequence  RotationAngleUnits=deg  RotationStandardAxis=+Z  RotationAngle=0.0  RotationArbitraryAxis=[0 0 1]  FollAlignAxisA=+X  BaseAlignAxisA=+Y  FollAlignAxisB=+Y  BaseAlignAxisB=+Z  RotationSequenceAxes=FollowerAxes  RotationSequence=XYZ  RotationSequenceAngles=smbData.link_active(4).Left.RigidTransform.angles  RotationSequenceAnglesUnits=rad  RotationMatrix=[1 0 0; 0 1 0; 0 0 1]
  Rigid Transform5 : sm_lib/Frames and Transforms/Rigid Transform  TranslationMethod=Cartesian  TranslationStandardOffset=0  TranslationLengthUnit=mm  TranslationStandardAxis=+Z  TranslationCartesianOffset=smbData.link_active(4).Right.RigidTransform.translation  TranslationROffset=0  TranslationROffsetUnits=m  TranslationZOffset=0  TranslationZOffsetUnits=m  TranslationThetaOffset=0  TranslationThetaOffsetUnits=deg  RotationMethod=RotationSequence  RotationAngleUnits=deg  RotationStandardAxis=+X  RotationAngle=90.0  RotationArbitraryAxis=[0 0 1]  FollAlignAxisA=+X  BaseAlignAxisA=+Y  FollAlignAxisB=+Y  BaseAlignAxisB=+Z  RotationSequenceAxes=FollowerAxes  RotationSequence=XYZ  RotationSequenceAngles=smbData.link_active(4).Right.RigidTransform.angles  RotationSequenceAnglesUnits=rad  RotationMatrix=[1 0 0; 0 1 0; 0 0 1]
  link_active_servomotion : sm_lib/Body Elements/File Solid  ExtGeomFileName=meshes\link_active_servomotion.STEP  UnitType=FromFile  ExtGeomFileUnits=m  StepReaderType=HEX  ExportEntireGeometry=off  InertiaType=Custom  Mass=smiData.link_active_servomotion.mass  MassUnits=kg  CenterOfMass=smiData.link_active_servomotion.CoM  CenterOfMassUnits=m  MomentsOfInertia=smiData.link_active_servomotion.MoI  MomentsOfInertiaUnits=kg*m^2  ProductsOfInertia=smiData.link_active_servomotion.PoI  ProductsOfInertiaUnits=kg*m^2  BasedOnType=Density  Density=1000  DensityUnits=kg/m^3  DoExposeReferenceFrame=on  SerializedFrames=<Frames/>  GraphicType=FromGeometry  MarkerShape=Sphere  MarkerSize=10  GraphicVisPropType=SimpleVisualProperties  GraphicDiffuseColor=smiData.link_active_servomotion.color  GraphicSpecularColor=[0.5 0.5 0.5 1.0]  GraphicAmbientColor=[0.15 0.15 0.15 1.0]  GraphicEmissiveColor=[0.0 0.0 0.0 1.0]  GraphicShininess=75  GraphicOpacity=smiData.link_active_servomotion.opacity
  Conn1 : PMIOPort  Side=Left
  Conn2 : PMIOPort  Port=2  Side=Right
  connections:
  Rigid Transform5/LConn1 -- Rigid Transform/RConn1 -- link_active_servomotion/RConn1
  Rigid Transform/LConn1 -- Conn1/RConn1
  Conn2/RConn1 -- Rigid Transform5/RConn1

== system stewartplatform/Model of Parallel Robot/Active Link5 ==
  Rigid Transform : sm_lib/Frames and Transforms/Rigid Transform  TranslationMethod=None  TranslationStandardOffset=0  TranslationLengthUnit=m  TranslationStandardAxis=+Z  TranslationCartesianOffset=[0 0 0]  TranslationROffset=0  TranslationROffsetUnits=m  TranslationZOffset=0  TranslationZOffsetUnits=m  TranslationThetaOffset=0  TranslationThetaOffsetUnits=deg  RotationMethod=RotationSequence  RotationAngleUnits=deg  RotationStandardAxis=+Z  RotationAngle=0.0  RotationArbitraryAxis=[0 0 1]  FollAlignAxisA=+X  BaseAlignAxisA=+Y  FollAlignAxisB=+Y  BaseAlignAxisB=+Z  RotationSequenceAxes=FollowerAxes  RotationSequence=XYZ  RotationSequenceAngles=smbData.link_active(5).Left.RigidTransform.angles  RotationSequenceAnglesUnits=rad  RotationMatrix=[1 0 0; 0 1 0; 0 0 1]
  Rigid Transform5 : sm_lib/Frames and Transforms/Rigid Transform  TranslationMethod=Cartesian  TranslationStandardOffset=0  TranslationLengthUnit=mm  TranslationStandardAxis=+Z  TranslationCartesianOffset=smbData.link_active(5).Right.RigidTransform.translation  TranslationROffset=0  TranslationROffsetUnits=m  TranslationZOffset=0  TranslationZOffsetUnits=m  TranslationThetaOffset=0  TranslationThetaOffsetUnits=deg  RotationMethod=RotationSequence  RotationAngleUnits=deg  RotationStandardAxis=+X  RotationAngle=90.0  RotationArbitraryAxis=[0 0 1]  FollAlignAxisA=+X  BaseAlignAxisA=+Y  FollAlignAxisB=+Y  BaseAlignAxisB=+Z  RotationSequenceAxes=FollowerAxes  RotationSequence=XYZ  RotationSequenceAngles=smbData.link_active(5).Right.RigidTransform.angles  RotationSequenceAnglesUnits=rad  RotationMatrix=[1 0 0; 0 1 0; 0 0 1]
  link_active_servomotion : sm_lib/Body Elements/File Solid  ExtGeomFileName=meshes\link_active_servomotion.STEP  UnitType=FromFile  ExtGeomFileUnits=m  StepReaderType=HEX  ExportEntireGeometry=off  InertiaType=Custom  Mass=smiData.link_active_servomotion.mass  MassUnits=kg  CenterOfMass=smiData.link_active_servomotion.CoM  CenterOfMassUnits=m  MomentsOfInertia=smiData.link_active_servomotion.MoI  MomentsOfInertiaUnits=kg*m^2  ProductsOfInertia=smiData.link_active_servomotion.PoI  ProductsOfInertiaUnits=kg*m^2  BasedOnType=Density  Density=1000  DensityUnits=kg/m^3  DoExposeReferenceFrame=on  SerializedFrames=<Frames/>  GraphicType=FromGeometry  MarkerShape=Sphere  MarkerSize=10  GraphicVisPropType=SimpleVisualProperties  GraphicDiffuseColor=smiData.link_active_servomotion.color  GraphicSpecularColor=[0.5 0.5 0.5 1.0]  GraphicAmbientColor=[0.15 0.15 0.15 1.0]  GraphicEmissiveColor=[0.0 0.0 0.0 1.0]  GraphicShininess=75  GraphicOpacity=smiData.link_active_servomotion.opacity
  Conn1 : PMIOPort  Side=Left
  Conn2 : PMIOPort  Port=2  Side=Right
  connections:
  Rigid Transform5/LConn1 -- Rigid Transform/RConn1 -- link_active_servomotion/RConn1
  Rigid Transform/LConn1 -- Conn1/RConn1
  Conn2/RConn1 -- Rigid Transform5/RConn1

== system stewartplatform/Model of Parallel Robot/Active Link6 ==
  Rigid Transform : sm_lib/Frames and Transforms/Rigid Transform  TranslationMethod=None  TranslationStandardOffset=0  TranslationLengthUnit=m  TranslationStandardAxis=+Z  TranslationCartesianOffset=[0 0 0]  TranslationROffset=0  TranslationROffsetUnits=m  TranslationZOffset=0  TranslationZOffsetUnits=m  TranslationThetaOffset=0  TranslationThetaOffsetUnits=deg  RotationMethod=RotationSequence  RotationAngleUnits=deg  RotationStandardAxis=+Z  RotationAngle=0.0  RotationArbitraryAxis=[0 0 1]  FollAlignAxisA=+X  BaseAlignAxisA=+Y  FollAlignAxisB=+Y  BaseAlignAxisB=+Z  RotationSequenceAxes=FollowerAxes  RotationSequence=XYZ  RotationSequenceAngles=smbData.link_active(6).Left.RigidTransform.angles  RotationSequenceAnglesUnits=rad  RotationMatrix=[1 0 0; 0 1 0; 0 0 1]
  Rigid Transform5 : sm_lib/Frames and Transforms/Rigid Transform  TranslationMethod=Cartesian  TranslationStandardOffset=0  TranslationLengthUnit=mm  TranslationStandardAxis=+Z  TranslationCartesianOffset=smbData.link_active(6).Right.RigidTransform.translation  TranslationROffset=0  TranslationROffsetUnits=m  TranslationZOffset=0  TranslationZOffsetUnits=m  TranslationThetaOffset=0  TranslationThetaOffsetUnits=deg  RotationMethod=RotationSequence  RotationAngleUnits=deg  RotationStandardAxis=+X  RotationAngle=90.0  RotationArbitraryAxis=[0 0 1]  FollAlignAxisA=+X  BaseAlignAxisA=+Y  FollAlignAxisB=+Y  BaseAlignAxisB=+Z  RotationSequenceAxes=FollowerAxes  RotationSequence=XYZ  RotationSequenceAngles=smbData.link_active(6).Right.RigidTransform.angles  RotationSequenceAnglesUnits=rad  RotationMatrix=[1 0 0; 0 1 0; 0 0 1]
  link_active_servomotion : sm_lib/Body Elements/File Solid  ExtGeomFileName=meshes\link_active_servomotion.STEP  UnitType=FromFile  ExtGeomFileUnits=m  StepReaderType=HEX  ExportEntireGeometry=off  InertiaType=Custom  Mass=smiData.link_active_servomotion.mass  MassUnits=kg  CenterOfMass=smiData.link_active_servomotion.CoM  CenterOfMassUnits=m  MomentsOfInertia=smiData.link_active_servomotion.MoI  MomentsOfInertiaUnits=kg*m^2  ProductsOfInertia=smiData.link_active_servomotion.PoI  ProductsOfInertiaUnits=kg*m^2  BasedOnType=Density  Density=1000  DensityUnits=kg/m^3  DoExposeReferenceFrame=on  SerializedFrames=<Frames/>  GraphicType=FromGeometry  MarkerShape=Sphere  MarkerSize=10  GraphicVisPropType=SimpleVisualProperties  GraphicDiffuseColor=smiData.link_active_servomotion.color  GraphicSpecularColor=[0.5 0.5 0.5 1.0]  GraphicAmbientColor=[0.15 0.15 0.15 1.0]  GraphicEmissiveColor=[0.0 0.0 0.0 1.0]  GraphicShininess=75  GraphicOpacity=smiData.link_active_servomotion.opacity
  Conn1 : PMIOPort  Side=Left
  Conn2 : PMIOPort  Port=2  Side=Right
  connections:
  Rigid Transform5/LConn1 -- Rigid Transform/RConn1 -- link_active_servomotion/RConn1
  Rigid Transform/LConn1 -- Conn1/RConn1
  Conn2/RConn1 -- Rigid Transform5/RConn1

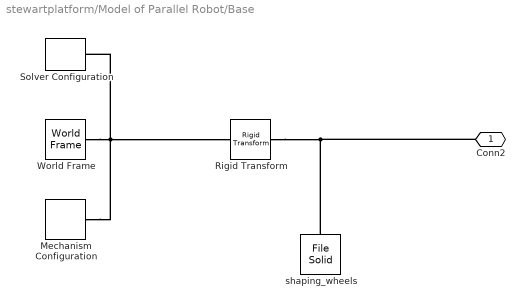
== system stewartplatform/Model of Parallel Robot/Base ==
  Mechanism Configuration : sm_lib/Utilities/Mechanism Configuration  UniformGravity=Constant  GravityVector=[0 0 -9.80665]  GravityUnits=m/s^2  LinearizationDelta=0.001
  Rigid Transform : sm_lib/Frames and Transforms/Rigid Transform  TranslationMethod=None  TranslationStandardOffset=0  TranslationLengthUnit=mm  TranslationStandardAxis=+Z  TranslationCartesianOffset=[0.0 0.0 -45.5]  TranslationROffset=0  TranslationROffsetUnits=m  TranslationZOffset=0  TranslationZOffsetUnits=m  TranslationThetaOffset=0  TranslationThetaOffsetUnits=deg  RotationMethod=RotationSequence  RotationAngleUnits=deg  RotationStandardAxis=+Z  RotationAngle=0.0  RotationArbitraryAxis=[0 0 1]  FollAlignAxisA=+X  BaseAlignAxisA=+Y  FollAlignAxisB=+Y  BaseAlignAxisB=+Z  RotationSequenceAxes=FollowerAxes  RotationSequence=XYZ  RotationSequenceAngles=smbData.shaping_wheels.Left.RigidTransform.angles  RotationSequenceAnglesUnits=rad  RotationMatrix=[1 0 0; 0 1 0; 0 0 1]
  Solver Configuration : nesl_utility/Solver Configuration  PhysicalDomain=network_engine_domain  SubClassName=solver  LeftPortType=input  RightPortType=generic  Tones=[]  Harmonics=[]  SimulateNoise=off  Profile=off  UseLocalSampling=off  EnableSwitchedLinearOptims=on  FrequencyDomain=off  UseCCode=off  RelTol=0.001  AbsTol=1e-06  MinStep=1e-09  ToWorkspace=off  RevertToSquareIcSolve=off  NumHomotopyIterations=100  PhasorMode=off  PhasorModeNumHarmonics=1  DoDC=off  ResidualTolerance=1e-09  UseLocalSolver=off  LocalSolverChoice=NE_BACKWARD_EULER_ADVANCER  LocalSolverSampleTime=0.001  DoFixedCost=off  MaxNonlinIter=3  MaxModeIter=2  LinearAlgebra=Sparse  EquationFormulation=NE_TIME_EF  DelaysMemoryBudget=1024  AutomaticFiltering=on  FilteringTimeConstant=0.001  PartitionStorageMethod=AS_NEEDED  PartitionMemoryBudget=1024  PartitionMethod=FAST
  World Frame : sm_lib/Frames and Transforms/World Frame
  shaping_wheels : sm_lib/Body Elements/File Solid  ExtGeomFileName=meshes\shaping_wheels.STEP  UnitType=FromFile  ExtGeomFileUnits=m  StepReaderType=HEX  ExportEntireGeometry=off  InertiaType=Custom  Mass=smiData.shaping_wheels.mass  MassUnits=kg  CenterOfMass=smiData.shaping_wheels.CoM  CenterOfMassUnits=m  MomentsOfInertia=smiData.shaping_wheels.MoI  MomentsOfInertiaUnits=kg*m^2  ProductsOfInertia=smiData.shaping_wheels.PoI  ProductsOfInertiaUnits=kg*m^2  BasedOnType=Density  Density=1000  DensityUnits=kg/m^3  DoExposeReferenceFrame=on  SerializedFrames=<Frames/>  GraphicType=FromGeometry  MarkerShape=Sphere  MarkerSize=10  GraphicVisPropType=SimpleVisualProperties  GraphicDiffuseColor=smiData.shaping_wheels.color  GraphicSpecularColor=[0.5 0.5 0.5 1.0]  GraphicAmbientColor=[0.15 0.15 0.15 1.0]  GraphicEmissiveColor=[0.0 0.0 0.0 1.0]  GraphicShininess=75  GraphicOpacity=smiData.shaping_wheels.opacity
  Conn2 : PMIOPort  Side=Right
  connections:
  shaping_wheels/RConn1 -- Conn2/RConn1 -- Rigid Transform/RConn1
  World Frame/RConn1 -- Rigid Transform/LConn1 -- Solver Configuration/RConn1 -- Mechanism Configuration/RConn1

== system stewartplatform/Model of Parallel Robot/Passive Link1 ==
  Passive_Link : sm_lib/Body Elements/File Solid  ExtGeomFileName=meshes\link_passive.STEP  UnitType=FromFile  ExtGeomFileUnits=m  StepReaderType=HEX  ExportEntireGeometry=off  InertiaType=Custom  Mass=smiData.link_passive.mass  MassUnits=kg  CenterOfMass=smiData.link_passive.CoM  CenterOfMassUnits=m  MomentsOfInertia=smiData.link_passive.MoI  MomentsOfInertiaUnits=kg*m^2  ProductsOfInertia=smiData.link_passive.PoI  ProductsOfInertiaUnits=kg*m^2  BasedOnType=Density  Density=1000  DensityUnits=kg/m^3  DoExposeReferenceFrame=on  SerializedFrames=<Frames/>  GraphicType=FromGeometry  MarkerShape=Sphere  MarkerSize=10  GraphicVisPropType=SimpleVisualProperties  GraphicDiffuseColor=smiData.link_passive.color  GraphicSpecularColor=[0.5 0.5 0.5 1.0]  GraphicAmbientColor=[0.15 0.15 0.15 1.0]  GraphicEmissiveColor=[0.0 0.0 0.0 1.0]  GraphicShininess=75  GraphicOpacity=smiData.link_passive.opacity
  Rigid Transform1 : sm_lib/Frames and Transforms/Rigid Transform  TranslationMethod=Cartesian  TranslationStandardOffset=0  TranslationLengthUnit=mm  TranslationStandardAxis=+Z  TranslationCartesianOffset=smbData.joint_spherical(1).Left.RigidTransform.translation  TranslationROffset=0  TranslationROffsetUnits=m  TranslationZOffset=0  TranslationZOffsetUnits=m  TranslationThetaOffset=0  TranslationThetaOffsetUnits=deg  RotationMethod=None  RotationAngleUnits=deg  RotationStandardAxis=+X  RotationAngle=90.0  RotationArbitraryAxis=[0 0 1]  FollAlignAxisA=+X  BaseAlignAxisA=+Y  FollAlignAxisB=+Y  BaseAlignAxisB=+Z  RotationSequenceAxes=FollowerAxes  RotationSequence=XYX  RotationSequenceAngles=[0 0 0]  RotationSequenceAnglesUnits=deg  RotationMatrix=[1 0 0; 0 1 0; 0 0 1]
  Spherical Joint : sm_lib/Joints/Spherical Joint  JointMode=Normal  SenseConstraintForce=off  SenseConstraintForceX=off  SenseConstraintForceY=off  SenseConstraintForceZ=off  SenseConstraintTorque=off  SenseConstraintTorqueX=off  SenseConstraintTorqueY=off  SenseConstraintTorqueZ=off  SenseTotalForce=off  SenseTotalForceX=off  SenseTotalForceY=off  SenseTotalForceZ=off  SenseTotalTorque=off  SenseTotalTorqueX=off  SenseTotalTorqueY=off  SenseTotalTorqueZ=off  CompositeWrenchDir=FollowerOnBase  CompositeWrenchFrame=BaseFrame  DefPosRotationMethod=None  DefPosRotationAngleUnits=deg  DefPosRotationStandardAxis=+Z  DefPosRotationAngle=0.0  DefPosRotationArbitraryAxis=[0 0 1]  DefPosFollAlignAxisA=+X  DefPosBaseAlignAxisA=+Y  DefPosFollAlignAxisB=+Y  DefPosBaseAlignAxisB=+Z  DefPosRotationSequenceAxes=FollowerAxes  DefPosRotationSequence=XYX  DefPosRotationSequenceAngles=[0 0 0]  DefPosRotationSequenceAnglesUnits=deg  DefPosRotationMatrix=[1 0 0; 0 1 0; 0 0 1]  EqPosRotationMethod=None  EqPosRotationAngleUnits=deg  EqPosRotationStandardAxis=+Z  EqPosRotationAngle=0.0  EqPosRotationArbitraryAxis=[0 0 1]  EqPosFollAlignAxisA=+X  EqPosBaseAlignAxisA=+Y  EqPosFollAlignAxisB=+Y  EqPosBaseAlignAxisB=+Z  EqPosRotationSequenceAxes=FollowerAxes  EqPosRotationSequence=XYX  EqPosRotationSequenceAngles=[0 0 0]  EqPosRotationSequenceAnglesUnits=deg  EqPosRotationMatrix=[1 0 0; 0 1 0; 0 0 1]  SpringStiffness=0  SpringStiffnessUnits=N*m/deg  DampingCoefficient=0  DampingCoefficientUnits=N*m/(deg/s)  ActuateTorqueX=off  ActuateTorqueY=off  ActuateTorqueZ=off  ActuateTorque=off  TorqueActuationMode=NoTorque  MotionActuationMode=ComputedMotion  ActuationFrame=BaseFrame  SensePosition=off  SenseVelocityX=off  SenseVelocityY=off  SenseVelocityZ=off  SenseVelocity=off  SenseAccelerationX=off  SenseAccelerationY=off  SenseAccelerationZ=off  SenseAcceleration=off  SenseTorqueX=off  SenseTorqueY=off  SenseTorqueZ=off  SenseTorqueForce=off  SenseLowerLimitTorqueMag=off  SenseUpperLimitTorqueMag=off  SensingFrame=BaseFrame  LowerLimitSpecify=off  LowerLimitBound=15  LowerLimitBoundUnits=deg  LowerLimitStiffness=1e4  LowerLimitStiffnessUnits=N*m/deg  LowerLimitDamping=10  LowerLimitDampingUnits=N*m/(deg/s)  LowerLimitTransitionRegionWidth=0.1  LowerLimitTransitionRegionWidthUnits=deg  UpperLimitSpecify=off  UpperLimitBound=45  UpperLimitBoundUnits=deg  UpperLimitStiffness=1e4  UpperLimitStiffnessUnits=N*m/deg  UpperLimitDamping=10  UpperLimitDampingUnits=N*m/(deg/s)  UpperLimitTransitionRegionWidth=0.1  UpperLimitTransitionRegionWidthUnits=deg  PositionTargetRotationMethod=None  PositionTargetRotationAngleUnits=deg  PositionTargetRotationStandardAxis=+Z  PositionTargetRotationAngle=0.0  PositionTargetRotationArbitraryAxis=[0 0 1]  PositionTargetFollAlignAxisA=+X  PositionTargetBaseAlignAxisA=+Y  PositionTargetFollAlignAxisB=+Y  PositionTargetBaseAlignAxisB=+Z  PositionTargetRotationSequenceAxes=FollowerAxes  PositionTargetRotationSequence=XYX  PositionTargetRotationSequenceAngles=[0 0 0]  PositionTargetRotationSequenceAnglesUnits=deg  PositionTargetRotationMatrix=[1 0 0; 0 1 0; 0 0 1]  PositionTargetSpecify=off  PositionTargetPriority=High  VelocityTargetValue=[0 0 0]  VelocityTargetValueUnits=deg/s  VelocityTargetSpecify=off  VelocityTargetPriority=High  VelocityTargetInFollowerFrame=on
  Spherical_Joint : sm_lib/Body Elements/File Solid  ExtGeomFileName=meshes\joint_spherical.STEP  UnitType=FromFile  ExtGeomFileUnits=m  StepReaderType=HEX  ExportEntireGeometry=off  InertiaType=Custom  Mass=smiData.joint_spherical.mass  MassUnits=kg  CenterOfMass=smiData.joint_spherical.CoM  CenterOfMassUnits=m  MomentsOfInertia=smiData.joint_spherical.MoI  MomentsOfInertiaUnits=kg*m^2  ProductsOfInertia=smiData.joint_spherical.PoI  ProductsOfInertiaUnits=kg*m^2  BasedOnType=Density  Density=1000  DensityUnits=kg/m^3  DoExposeReferenceFrame=on  SerializedFrames=<Frames/>  GraphicType=FromGeometry  MarkerShape=Sphere  MarkerSize=10  GraphicVisPropType=SimpleVisualProperties  GraphicDiffuseColor=smiData.joint_spherical.color  GraphicSpecularColor=[0.5 0.5 0.5 1.0]  GraphicAmbientColor=[0.15 0.15 0.15 1.0]  GraphicEmissiveColor=[0.0 0.0 0.0 1.0]  GraphicShininess=75  GraphicOpacity=smiData.joint_spherical.opacity
  Conn1 : PMIOPort  Side=Left
  Conn2 : PMIOPort  Port=2  Side=Right
  connections:
  Spherical_Joint/RConn1 -- Spherical Joint/LConn1 -- Rigid Transform1/RConn1
  Rigid Transform1/LConn1 -- Conn1/RConn1 -- Passive_Link/RConn1
  Spherical Joint/RConn1 -- Conn2/RConn1

== system stewartplatform/Model of Parallel Robot/Passive Link2 ==
  Passive_Link : sm_lib/Body Elements/File Solid  ExtGeomFileName=meshes\link_passive.STEP  UnitType=FromFile  ExtGeomFileUnits=m  StepReaderType=HEX  ExportEntireGeometry=off  InertiaType=Custom  Mass=smiData.link_passive.mass  MassUnits=kg  CenterOfMass=smiData.link_passive.CoM  CenterOfMassUnits=m  MomentsOfInertia=smiData.link_passive.MoI  MomentsOfInertiaUnits=kg*m^2  ProductsOfInertia=smiData.link_passive.PoI  ProductsOfInertiaUnits=kg*m^2  BasedOnType=Density  Density=1000  DensityUnits=kg/m^3  DoExposeReferenceFrame=on  SerializedFrames=<Frames/>  GraphicType=FromGeometry  MarkerShape=Sphere  MarkerSize=10  GraphicVisPropType=SimpleVisualProperties  GraphicDiffuseColor=smiData.link_passive.color  GraphicSpecularColor=[0.5 0.5 0.5 1.0]  GraphicAmbientColor=[0.15 0.15 0.15 1.0]  GraphicEmissiveColor=[0.0 0.0 0.0 1.0]  GraphicShininess=75  GraphicOpacity=smiData.link_passive.opacity
  Rigid Transform1 : sm_lib/Frames and Transforms/Rigid Transform  TranslationMethod=Cartesian  TranslationStandardOffset=0  TranslationLengthUnit=mm  TranslationStandardAxis=+Z  TranslationCartesianOffset=smbData.joint_spherical(2).Left.RigidTransform.translation  TranslationROffset=0  TranslationROffsetUnits=m  TranslationZOffset=0  TranslationZOffsetUnits=m  TranslationThetaOffset=0  TranslationThetaOffsetUnits=deg  RotationMethod=None  RotationAngleUnits=deg  RotationStandardAxis=+X  RotationAngle=90.0  RotationArbitraryAxis=[0 0 1]  FollAlignAxisA=+X  BaseAlignAxisA=+Y  FollAlignAxisB=+Y  BaseAlignAxisB=+Z  RotationSequenceAxes=FollowerAxes  RotationSequence=XYX  RotationSequenceAngles=[0 0 0]  RotationSequenceAnglesUnits=deg  RotationMatrix=[1 0 0; 0 1 0; 0 0 1]
  Spherical Joint : sm_lib/Joints/Spherical Joint  JointMode=Normal  SenseConstraintForce=off  SenseConstraintForceX=off  SenseConstraintForceY=off  SenseConstraintForceZ=off  SenseConstraintTorque=off  SenseConstraintTorqueX=off  SenseConstraintTorqueY=off  SenseConstraintTorqueZ=off  SenseTotalForce=off  SenseTotalForceX=off  SenseTotalForceY=off  SenseTotalForceZ=off  SenseTotalTorque=off  SenseTotalTorqueX=off  SenseTotalTorqueY=off  SenseTotalTorqueZ=off  CompositeWrenchDir=FollowerOnBase  CompositeWrenchFrame=BaseFrame  DefPosRotationMethod=None  DefPosRotationAngleUnits=deg  DefPosRotationStandardAxis=+Z  DefPosRotationAngle=0.0  DefPosRotationArbitraryAxis=[0 0 1]  DefPosFollAlignAxisA=+X  DefPosBaseAlignAxisA=+Y  DefPosFollAlignAxisB=+Y  DefPosBaseAlignAxisB=+Z  DefPosRotationSequenceAxes=FollowerAxes  DefPosRotationSequence=XYX  DefPosRotationSequenceAngles=[0 0 0]  DefPosRotationSequenceAnglesUnits=deg  DefPosRotationMatrix=[1 0 0; 0 1 0; 0 0 1]  EqPosRotationMethod=None  EqPosRotationAngleUnits=deg  EqPosRotationStandardAxis=+Z  EqPosRotationAngle=0.0  EqPosRotationArbitraryAxis=[0 0 1]  EqPosFollAlignAxisA=+X  EqPosBaseAlignAxisA=+Y  EqPosFollAlignAxisB=+Y  EqPosBaseAlignAxisB=+Z  EqPosRotationSequenceAxes=FollowerAxes  EqPosRotationSequence=XYX  EqPosRotationSequenceAngles=[0 0 0]  EqPosRotationSequenceAnglesUnits=deg  EqPosRotationMatrix=[1 0 0; 0 1 0; 0 0 1]  SpringStiffness=0  SpringStiffnessUnits=N*m/deg  DampingCoefficient=0  DampingCoefficientUnits=N*m/(deg/s)  ActuateTorqueX=off  ActuateTorqueY=off  ActuateTorqueZ=off  ActuateTorque=off  TorqueActuationMode=NoTorque  MotionActuationMode=ComputedMotion  ActuationFrame=BaseFrame  SensePosition=off  SenseVelocityX=off  SenseVelocityY=off  SenseVelocityZ=off  SenseVelocity=off  SenseAccelerationX=off  SenseAccelerationY=off  SenseAccelerationZ=off  SenseAcceleration=off  SenseTorqueX=off  SenseTorqueY=off  SenseTorqueZ=off  SenseTorqueForce=off  SenseLowerLimitTorqueMag=off  SenseUpperLimitTorqueMag=off  SensingFrame=BaseFrame  LowerLimitSpecify=off  LowerLimitBound=15  LowerLimitBoundUnits=deg  LowerLimitStiffness=1e4  LowerLimitStiffnessUnits=N*m/deg  LowerLimitDamping=10  LowerLimitDampingUnits=N*m/(deg/s)  LowerLimitTransitionRegionWidth=0.1  LowerLimitTransitionRegionWidthUnits=deg  UpperLimitSpecify=off  UpperLimitBound=45  UpperLimitBoundUnits=deg  UpperLimitStiffness=1e4  UpperLimitStiffnessUnits=N*m/deg  UpperLimitDamping=10  UpperLimitDampingUnits=N*m/(deg/s)  UpperLimitTransitionRegionWidth=0.1  UpperLimitTransitionRegionWidthUnits=deg  PositionTargetRotationMethod=None  PositionTargetRotationAngleUnits=deg  PositionTargetRotationStandardAxis=+Z  PositionTargetRotationAngle=0.0  PositionTargetRotationArbitraryAxis=[0 0 1]  PositionTargetFollAlignAxisA=+X  PositionTargetBaseAlignAxisA=+Y  PositionTargetFollAlignAxisB=+Y  PositionTargetBaseAlignAxisB=+Z  PositionTargetRotationSequenceAxes=FollowerAxes  PositionTargetRotationSequence=XYX  PositionTargetRotationSequenceAngles=[0 0 0]  PositionTargetRotationSequenceAnglesUnits=deg  PositionTargetRotationMatrix=[1 0 0; 0 1 0; 0 0 1]  PositionTargetSpecify=off  PositionTargetPriority=High  VelocityTargetValue=[0 0 0]  VelocityTargetValueUnits=deg/s  VelocityTargetSpecify=off  VelocityTargetPriority=High  VelocityTargetInFollowerFrame=on
  Spherical_Joint : sm_lib/Body Elements/File Solid  ExtGeomFileName=meshes\joint_spherical.STEP  UnitType=FromFile  ExtGeomFileUnits=m  StepReaderType=HEX  ExportEntireGeometry=off  InertiaType=Custom  Mass=smiData.joint_spherical.mass  MassUnits=kg  CenterOfMass=smiData.joint_spherical.CoM  CenterOfMassUnits=m  MomentsOfInertia=smiData.joint_spherical.MoI  MomentsOfInertiaUnits=kg*m^2  ProductsOfInertia=smiData.joint_spherical.PoI  ProductsOfInertiaUnits=kg*m^2  BasedOnType=Density  Density=1000  DensityUnits=kg/m^3  DoExposeReferenceFrame=on  SerializedFrames=<Frames/>  GraphicType=FromGeometry  MarkerShape=Sphere  MarkerSize=10  GraphicVisPropType=SimpleVisualProperties  GraphicDiffuseColor=smiData.joint_spherical.color  GraphicSpecularColor=[0.5 0.5 0.5 1.0]  GraphicAmbientColor=[0.15 0.15 0.15 1.0]  GraphicEmissiveColor=[0.0 0.0 0.0 1.0]  GraphicShininess=75  GraphicOpacity=smiData.joint_spherical.opacity
  Conn1 : PMIOPort  Side=Left
  Conn2 : PMIOPort  Port=2  Side=Right
  connections:
  Spherical Joint/LConn1 -- Spherical_Joint/RConn1 -- Rigid Transform1/RConn1
  Rigid Transform1/LConn1 -- Passive_Link/RConn1 -- Conn1/RConn1
  Conn2/RConn1 -- Spherical Joint/RConn1
